simulink library "centralAngle_ul"  (R2018b)
settings: Solver=VariableStepAuto  StartTime=0.0  StopTime=10.0  RelTol=1e-3
settings Model: Creator=James Reed  LastModifiedBy=James Reed

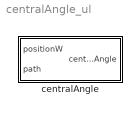
== system centralAngle_ul ==
  centralAngle : Subsystem

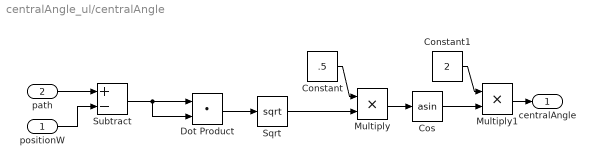
== system centralAngle_ul/centralAngle ==
  "positionW " : Inport
  "path " : Inport  Port=2
  Constant : Constant  Value=.5
  Constant1 : Constant  Value=2
  Cos : Trigonometry  Operator=asin
  Dot Product : DotProduct  InputSameDT=on  OutDataTypeStr=Inherit: Inherit via internal rule
  Multiply : Product
  Multiply1 : Product
  Sqrt : Sqrt  SaturateOnIntegerOverflow=on
  Subtract : Sum  Inputs=+-
  "centralAngle " : Outport
  wires:
  Dot Product/1 -> Sqrt/1
  Subtract/1 -> Dot Product/2, Dot Product/1
  Constant1/1 -> Multiply1/1
  Cos/1 -> Multiply1/2
  Multiply/1 -> Cos/1
  Sqrt/1 -> Multiply/2
  Multiply1/1 -> "centralAngle "/1
  "positionW "/1 -> Subtract/2
  Constant/1 -> Multiply/1
  "path "/1 -> Subtract/1
